simulink model "integrier_1"  (Simulink 5.0)
settings: Solver=ode45  StartTime=0.0  StopTime=10.0  RelTol=1e-3
libraries: dsparch4 x3, dspsigops x1
settings Model: Creator=svenhoffmann  LastModifiedBy=svenhoffmann  ExtModeAutoUpdateStatusClock=off

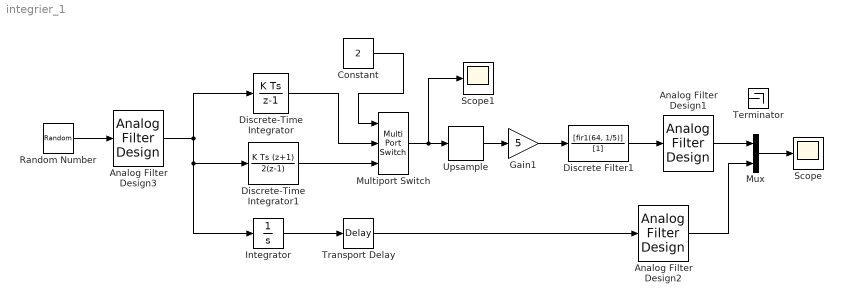
== system integrier_1 ==
  Analog Filter Design1 : dsparch4/Analog Filter Design  method=Butterworth  filttype=Lowpass  N=8  Wlo=2*pi*1000  Whi=80  Rp=2  Rs=40
  Analog Filter Design2 : dsparch4/Analog Filter Design  method=Butterworth  filttype=Lowpass  N=8  Wlo=2*pi*1000  Whi=80  Rp=2  Rs=40
  Analog Filter Design3 : dsparch4/Analog Filter Design  method=Butterworth  filttype=Lowpass  N=8  Wlo=2*pi*300  Whi=80  Rp=2  Rs=40
  Constant : Constant  Value=2
  Discrete Filter1 : DiscreteFilter  Numerator=[fir1(64, 1/5)]  Denominator=[1]  SampleTime=1/(5*1000)
  Discrete-Time Integrator : DiscreteIntegrator  SampleTime=1/1000
  Discrete-Time Integrator1 : DiscreteIntegrator  IntegratorMethod=Trapezoidal  SampleTime=1/1000
  Gain1 : Gain  Gain=5  SaturateOnIntegerOverflow=on
  Integrator : Integrator
  Multiport Switch : MultiPortSwitch  Inputs=2  SaturateOnIntegerOverflow=on
  Mux : Mux  Inputs=2
  Random Number : RandomNumber  SampleTime=0
  Scope : Scope
      settings: YMin=-0.035  YMax=0.005
  Scope1 : Scope
      settings: YMin=-0.009  YMax=0.006
  Terminator : Terminator
  Transport Delay : TransportDelay  DelayTime=7/1000
  Upsample : dspsigops/Upsample  N=5  phase=0  ic=0  mode=Maintain input frame size
  wires:
  Random Number/1 -> Analog Filter Design3/1
  Mux/1 -> Scope/1
  Constant/1 -> Multiport Switch/1
  Discrete-Time Integrator/1 -> Multiport Switch/2
  Integrator/1 -> Transport Delay/1
  Discrete-Time Integrator1/1 -> Multiport Switch/3
  Analog Filter Design3/1 -> Discrete-Time Integrator1/1, Integrator/1, Discrete-Time Integrator/1
  Analog Filter Design2/1 -> Mux/2
  Upsample/1 -> Gain1/1
  Gain1/1 -> Discrete Filter1/1
  Discrete Filter1/1 -> Analog Filter Design1/1
  Analog Filter Design1/1 -> Mux/1
  Multiport Switch/1 -> Upsample/1, Scope1/1
  Transport Delay/1 -> Analog Filter Design2/1
